simulink model "RotationalSpeedController"  (R2015b)
settings: Solver=VariableStepAuto  StartTime=0.0  StopTime=0.05  RelTol=1e-3
values from neighbouring files (symbols this model uses):
  Aplant = [0 1; 0 -K_fr/I]    [BaseParams.m]
  Bplant = [0; 1/I]    [BaseParams.m]
  Cplant = [0 1]    [BaseParams.m]
  Dact = [0.001 1]    [BaseParams.m]
  Dplant = [0]    [BaseParams.m]
  Ki = 26.5841    [BaseParams.m]
  Kp = 4.0289    [BaseParams.m]
  Nact = [1]    [BaseParams.m]
libraries: fl_lib x7, nesl_utility x4
settings Model: Creator=jje  LastModifiedBy=jje

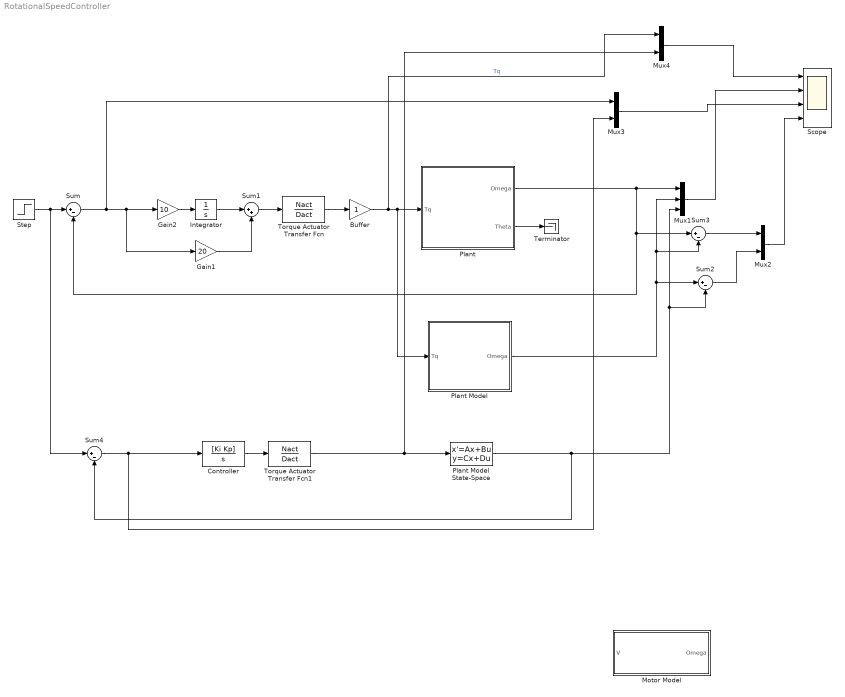
== system RotationalSpeedController ==
  Buffer : Gain
  Controller : TransferFcn  Numerator=[Ki Kp]  Denominator=[1 0]
  Gain1 : Gain  Gain=20
  Gain2 : Gain  Gain=10
  Integrator : Integrator
  Motor Model : Subsystem
  Mux1 : Mux  Inputs=3
  Mux2 : Mux  Inputs=2
  Mux3 : Mux  Inputs=2
  Mux4 : Mux  Inputs=2
  Plant : Subsystem
  Plant Model : Subsystem
  Plant Model State-Space : StateSpace  A=Aplant  B=Bplant  C=Cplant  D=Dplant  X0=0
  Scope : Scope  NumInputPorts=4
  Step : Step  Time=0.01  SampleTime=0
  Sum{,2..4} (4 alike) : Sum  Inputs=|+-
  Sum1 : Sum  Inputs=|++
  Terminator : Terminator
  Torque Actuator Transfer Fcn : TransferFcn  Numerator=Nact  Denominator=Dact
  Torque Actuator Transfer Fcn1 : TransferFcn  Numerator=Nact  Denominator=Dact
  wires:
  Buffer/1 -> Plant Model/1(Tq), Plant/1(Tq), Mux4/1  "Tq"
  Plant/1(Omega) -> Mux1/1, Sum3/1, Sum/2
  Integrator/1 -> Sum1/1
  Gain1/1 -> Sum1/2
  Sum/1 -> Mux3/1, Gain1/1, Gain2/1
  Gain2/1 -> Integrator/1
  Sum1/1 -> Torque Actuator Transfer Fcn/1
  Step/1 -> Sum4/1, Sum/1
  Torque Actuator Transfer Fcn/1 -> Buffer/1
  Plant/2(Theta) -> Terminator/1
  Mux1/1 -> Scope/2
  Plant Model/1(Omega) -> Sum2/1, Sum3/2, Mux1/2
  Plant Model State-Space/1 -> Sum2/2, Mux1/3, Sum4/2
  Mux2/1 -> Scope/4
  Sum3/1 -> Mux2/1
  Sum2/1 -> Mux2/2
  Controller/1 -> Torque Actuator Transfer Fcn1/1
  Torque Actuator Transfer Fcn1/1 -> Mux4/2, Plant Model State-Space/1
  Sum4/1 -> Controller/1, Mux3/2
  Mux3/1 -> Scope/3
  Mux4/1 -> Scope/1

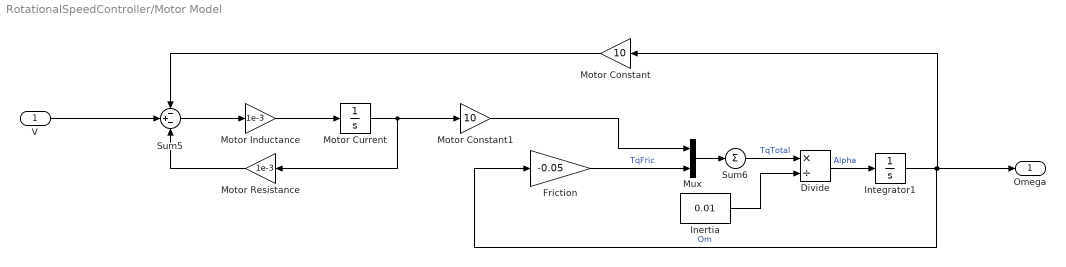
== system RotationalSpeedController/Motor Model ==
  V : Inport
  Divide : Product  Inputs=*/
  Friction : Gain  Gain=-0.05
  Inertia : Constant  Value=0.01
  Integrator1 : Integrator
  Motor Constant : Gain  Gain=10
  Motor Constant1 : Gain  Gain=10
  Motor Current : Integrator
  Motor Inductance : Gain  Gain=1e-3
  Motor Resistance : Gain  Gain=1e-3
  Mux : Mux  Inputs=2
  Sum5 : Sum  Inputs=-+-
  Sum6 : Sum  Inputs=1
  Omega : Outport
  wires:
  Motor Constant/1 -> Sum5/1
  Motor Constant1/1 -> Mux/1
  Motor Resistance/1 -> Sum5/3
  Sum6/1 -> Divide/1  "TqTotal"
  Integrator1/1 -> Omega/1, Motor Constant/1, Friction/1  "Om"
  Divide/1 -> Integrator1/1  "Alpha"
  Inertia/1 -> Divide/2
  Mux/1 -> Sum6/1
  Friction/1 -> Mux/2  "TqFric"
  V/1 -> Sum5/2
  Motor Inductance/1 -> Motor Current/1
  Sum5/1 -> Motor Inductance/1
  Motor Current/1 -> Motor Constant1/1, Motor Resistance/1

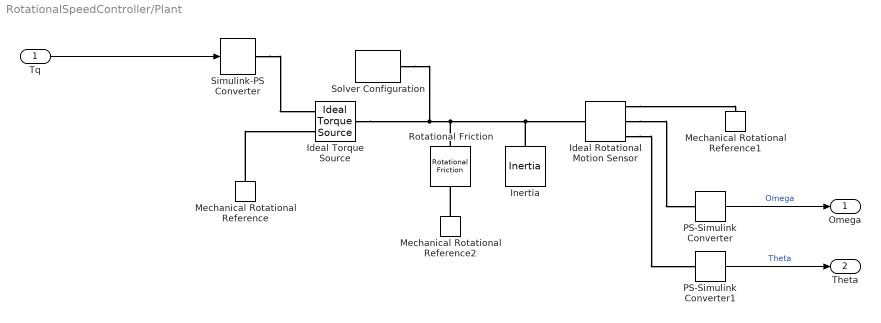
== system RotationalSpeedController/Plant ==
  Tq : Inport
  Ideal Rotational Motion Sensor : fl_lib/Mechanical/Mechanical Sensors/Ideal Rotational Motion Sensor  offset=0 rad
  Ideal Torque Source : fl_lib/Mechanical/Mechanical Sources/Ideal Torque Source
  Inertia : fl_lib/Mechanical/Rotational Elements/Inertia  inertia=0.01 kg*m^2  w_specify=off  w_priority=None  w=0 rad/s  t_specify=off  t_priority=None  t=0 N*m
      settings: AttributesFormatString=%<inertia>
  Mechanical Rotational Reference : fl_lib/Mechanical/Rotational Elements/Mechanical Rotational Reference
  Mechanical Rotational Reference1 : fl_lib/Mechanical/Rotational Elements/Mechanical Rotational Reference
  Mechanical Rotational Reference2 : fl_lib/Mechanical/Rotational Elements/Mechanical Rotational Reference
  PS-Simulink Converter : nesl_utility/PS-Simulink Converter  PhysicalDomain=network_engine_domain  SubClassName=ps_output  LeftPortType=input  RightPortType=output  PseudoPeriodic=off  Frequencies=[]  Unit=1  AffineConversion=off
  PS-Simulink Converter1 : nesl_utility/PS-Simulink Converter  PhysicalDomain=network_engine_domain  SubClassName=ps_output  LeftPortType=input  RightPortType=output  PseudoPeriodic=off  Frequencies=[]  Unit=1  AffineConversion=off
  Rotational Friction : fl_lib/Mechanical/Rotational Elements/Rotational Friction  brkwy_trq=0.1 N*m  Col_trq=0.001 N*m  visc_coef=0.05 N*m/(rad/s)  trans_coef=10 s/rad  vel_thr=1e-4 rad/s  w_specify=off  w_priority=None  w=0 rad/s  t_specify=off  t_priority=None  t=0 N*m
  Simulink-PS Converter : nesl_utility/Simulink-PS Converter  PhysicalDomain=network_engine_domain  SubClassName=ps_input  LeftPortType=input  RightPortType=output  PseudoPeriodic=off  Frequencies=[]  NoiseDistribution=none  NoiseParameters=[]  Unit=1  AffineConversion=off  InputFiltering=off  SimscapeFilterOrder=1  InputFilterTimeConstant=0.001  UdotUserProvided=1
  Solver Configuration : nesl_utility/Solver Configuration  PhysicalDomain=network_engine_domain  SubClassName=solver  LeftPortType=input  RightPortType=generic  Accelerate=off  Tones=[]  Harmonics=[]  SimulateNoise=off  Profile=off  UseLocalSampling=off  EnableSwitchedLinearOptims=on  FrequencyDomain=off  UseCCode=off  RelTol=0.001  AbsTol=1e-06  MinStep=1e-09  ToWorkspace=off  RevertToSquareIcSolve=off  NumHomotopyIterations=100  PhasorMode=off  PhasorModeNumHarmonics=1  DoDC=off  ResidualTolerance=1e-09  UseLocalSolver=off  LocalSolverChoice=NE_BACKWARD_EULER_ADVANCER  LocalSolverSampleTime=0.001  DoFixedCost=off  MaxNonlinIter=3  MaxModeIter=2  LinearAlgebra=Sparse  DelaysMemoryBudget=1024  AutomaticFiltering=on  FilteringTimeConstant=0.001
  Omega : Outport
  Theta : Outport  Port=2
  wires:
  Tq/1 -> Simulink-PS Converter/1
  PS-Simulink Converter/1 -> Omega/1  "Omega"
  PS-Simulink Converter1/1 -> Theta/1  "Theta"
  connections:
  Mechanical Rotational Reference/LConn1 -- Ideal Torque Source/RConn2
  Simulink-PS Converter/RConn1 -- Ideal Torque Source/RConn1
  Ideal Torque Source/LConn1 -- Solver Configuration/RConn1 -- Rotational Friction/LConn1 -- Inertia/LConn1 -- Ideal Rotational Motion Sensor/LConn1
  Ideal Rotational Motion Sensor/RConn2 -- PS-Simulink Converter/LConn1
  Ideal Rotational Motion Sensor/RConn3 -- PS-Simulink Converter1/LConn1
  Mechanical Rotational Reference2/LConn1 -- Rotational Friction/RConn1
  Ideal Rotational Motion Sensor/RConn1 -- Mechanical Rotational Reference1/LConn1

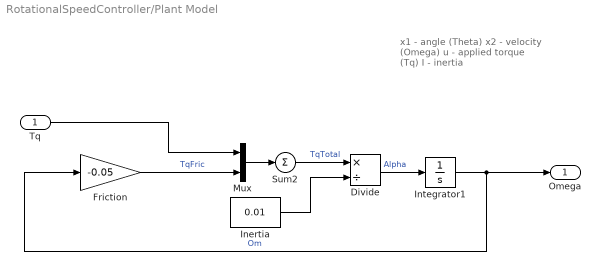
== system RotationalSpeedController/Plant Model ==
  note: x1 - angle (Theta)
      | x2 - velocity (Omega)
      | u - applied torque (Tq)
      | I - inertia
  Tq : Inport
  Divide : Product  Inputs=*/
  Friction : Gain  Gain=-0.05
  Inertia : Constant  Value=0.01
  Integrator1 : Integrator
  Mux : Mux  Inputs=2
  Sum2 : Sum  Inputs=1
  Omega : Outport
  wires:
  Tq/1 -> Mux/1
  Sum2/1 -> Divide/1  "TqTotal"
  Integrator1/1 -> Omega/1, Friction/1  "Om"
  Divide/1 -> Integrator1/1  "Alpha"
  Inertia/1 -> Divide/2
  Mux/1 -> Sum2/1
  Friction/1 -> Mux/2  "TqFric"
